simulink model "attiude_singularity"  (Simulink 6.0)
settings: Solver=ode45  StartTime=0.0  StopTime=4  MaxStep=0.001  RelTol=1e-5
undefined symbols (not defined in the file or in its folder): Euler, Quat, quat2euler
libraries: simulink x3
settings Model: LastModifiedBy=farrell
settings OptimizationCC: BooleanDataType=off
settings DebuggingCC: SolverPrmCheckMsg=none
settings HardwareCC: TargetUnknown=on
settings STFCustomTargetCC: TargetFcnLib=ansi_tfl_tmw.mat  GenFloatMathFcnCalls=ANSI_C  ModelReferenceCompliant=off  SystemTargetFile=grt.tlc

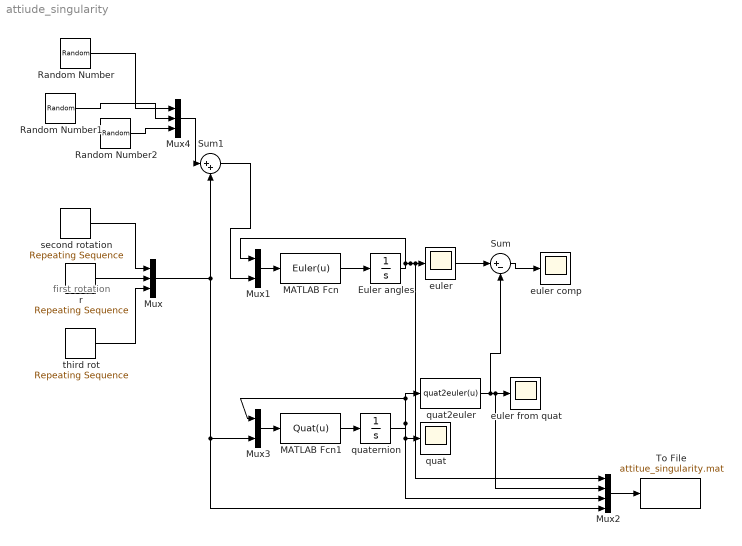
== system attiude_singularity ==
  note: first rotation
  Euler angles : Integrator
  MATLAB Fcn : MATLABFcn  MATLABFcn=Euler(u)  OutputDimensions=3
  MATLAB Fcn1 : MATLABFcn  MATLABFcn=Quat(u)  OutputDimensions=4
  Mux : Mux  Inputs=3
  Mux1 : Mux  Inputs=2
  Mux2 : Mux
  Mux3 : Mux  Inputs=2
  Mux4 : Mux  Inputs=3
  Random Number : RandomNumber  Variance=0.001  SampleTime=0
  Random Number1 : RandomNumber  Variance=0.001  SampleTime=0
  Random Number2 : RandomNumber  Variance=0.001  SampleTime=0
  Sum : Sum  Inputs=|+-  SaturateOnIntegerOverflow=on  InputSameDT=on
  Sum1 : Sum  Inputs=|++  SaturateOnIntegerOverflow=on  InputSameDT=on
  To File : ToFile  Filename=attitue_singularity.mat  MatrixName=dat  SampleTime=0.01
  euler : Scope
      settings: TimeRange=4  YMin=-1.5  YMax=2
  euler comp : Scope
      settings: TimeRange=4  YMax=4  SaveName=ScopeData3
  euler from quat : Scope
      settings: TimeRange=4  YMin=-4  YMax=4  SaveName=ScopeData2
  quat : Scope
      settings: TimeRange=4  YMin=-1  YMax=1.5
  quat2euler : MATLABFcn  MATLABFcn=quat2euler(u)  OutputDimensions=3
  quaternion : Integrator  InitialCondition=[1;zeros(3,1)]
  r : simulink/Sources/Repeating Sequence  rep_seq_t=[0 1 1.00000000001 4]  rep_seq_y="[pi/2  pi/2 0 0]"
  second rotation : simulink/Sources/Repeating Sequence  rep_seq_t=[0 1 1.000000001 2 2.0000000001 3 3.000000001 5]  rep_seq_y="[0 0 pi/2  pi/2 0 0 -pi/2 -pi/2 ]"
  third rot : simulink/Sources/Repeating Sequence  rep_seq_t=[0 2 2.00000000001 3 3.0000000000001 4]  rep_seq_y="[0 0 pi/2                      pi/2 0 0]"
  wires:
  Mux1/1 -> MATLAB Fcn/1
  Mux/1 -> Mux3/2, Mux2/4, Sum1/2
  MATLAB Fcn/1 -> Euler angles/1
  Euler angles/1 -> Mux1/1, euler/1, Sum/1, Mux2/1
  Mux3/1 -> MATLAB Fcn1/1
  MATLAB Fcn1/1 -> quaternion/1
  quaternion/1 -> quat2euler/1, Mux3/1, quat/1, Mux2/3
  quat2euler/1 -> Sum/2, euler from quat/1, Mux2/2
  Sum/1 -> euler comp/1
  r/1 -> Mux/2
  second rotation/1 -> Mux/1
  third rot/1 -> Mux/3
  Mux2/1 -> To File/1
  Random Number/1 -> Mux4/1
  Random Number1/1 -> Mux4/2
  Random Number2/1 -> Mux4/3
  Sum1/1 -> Mux1/2
  Mux4/1 -> Sum1/1
